simulink library "spsDiodeModel_R"  (R2023b)
settings: Solver=ode45  StartTime=0.0  StopTime=10.0  RelTol=1e-3
undefined symbols (not defined in the file): IC, Lon, Ron, Vf
settings Model: Creator=The MathWorks, Inc.  LastModifiedBy=rober
settings SolverCC: AlgebraicLoopSolver=TrustRegion
settings DataIOCC: LimitDataPoints=on  SaveFormat=Array  SignalLoggingSaveFormat=ModelDataLogs  ReturnWorkspaceOutputs=off
settings OptimizationCC: BlockReduction=off  BooleanDataType=off  ExpressionDepthLimit=2147483647  LifeSpan=inf
settings DebuggingCC: SaveWithParameterizedLinksMsg=none  UnderspecifiedInitializationDetection=Classic  MergeDetectMultiDrivingBlocksExec=none  SignalResolutionControl=TryResolveAllWithWarning  FcnCallInpInsideContextMsg=warning  UnconnectedInputMsg=warning  UnconnectedOutputMsg=warning  UnconnectedLineMsg=warning  StateNameClashWarn=warning  SFUnexpectedBacktrackingDiag=warning  SFNoUnconditionalDefaultTransitionDiag=warning  SFExecutionAtInitializationDiag=none  ArithmeticOperatorsInVariantConditions=warning
settings HardwareCC: ProdBitPerPointer=32  ProdBitPerSizeT=32  ProdBitPerPtrDiffT=32  ProdLargestAtomicFloat=None  ProdIntDivRoundTo=Undefined  ProdEndianess=Unspecified  ProdWordSize=32  ProdHWDeviceType=32-bit Generic  TargetUnknown=on
settings ModelReferenceCC: PropagateSignalLabelsOutOfModel=off
settings SFSimCC: SimUseLocalCustomCode=off  CustomCodeUndefinedFunction=UseInterfaceOnly
settings RTWCC: RTWUseLocalCustomCode=off
settings CodeAppCC: StateflowObjectComments=on
settings GRTTargetCC: TargetLangStandard=C89/C90 (ANSI)  CombineOutputUpdateFcns=off  GRTInterface=on
settings ConfigComp: CovMetricSettings=dw  CovSaveCumulativeToWorkspaceVar=on  CovSaveSingleToWorkspaceVar=on  CovExternalEMLEnable=off  CovSFcnEnable=off

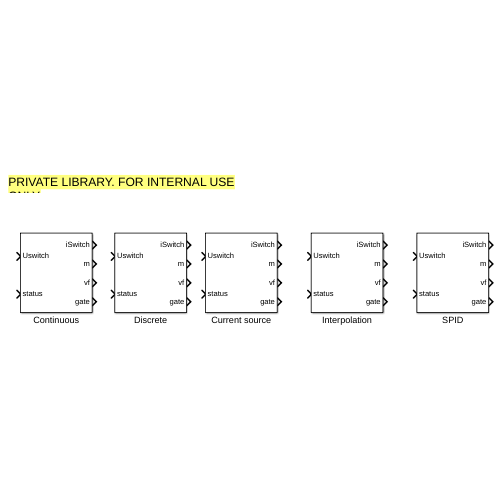
[thumbnail: Simulink's stored preview of the top-level diagram]
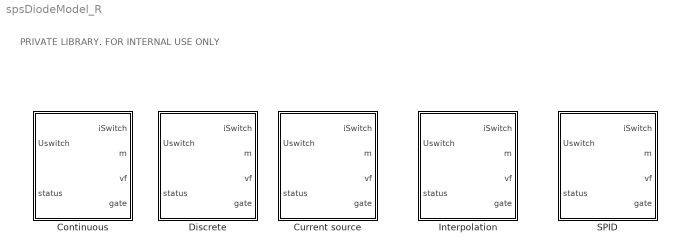
== system spsDiodeModel_R ==
  note: PRIVATE LIBRARY. FOR INTERNAL USE ONLY
  Continuous : Subsystem  mask(ContinuousModel){}
  Current source : Subsystem  mask(CurrentSourceDiode){}
  Discrete : Subsystem  mask(DiscreteModel){}
  Interpolation : Subsystem  mask(DiscreteModel){}
  SPID : Subsystem  mask(DiscreteModel){}

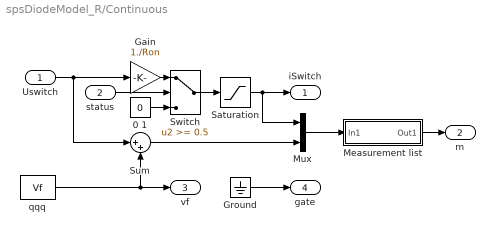
== system spsDiodeModel_R/Continuous ==
  Uswitch : Inport
  status : Inport  Port=2
  0 1 : Constant  Value=0
  Gain : Gain  Gain=1./Ron  SaturateOnIntegerOverflow=on  OutDataTypeStr=Inherit: Same as input  ParamDataTypeStr=Inherit: Same as input
  Ground : Ground
  Measurement list : Subsystem
  Mux : Mux  Inputs=2
  Saturation : Saturate  UpperLimit=inf  LowerLimit=0
  Sum : Sum  Inputs=|++  InputSameDT=on  SaturateOnIntegerOverflow=on  OutDataTypeStr=Inherit: Same as first input
  Switch : Switch  Threshold=0.5  SaturateOnIntegerOverflow=off
  qqq : Constant  Value=Vf
  iSwitch : Outport
  m : Outport  Port=2
  vf : Outport  Port=3
  gate : Outport  Port=4
  wires:
  Uswitch/1 -> Sum/1, Gain/1
  Gain/1 -> Switch/1
  0 1/1 -> Switch/3
  Switch/1 -> Saturation/1
  qqq/1 -> vf/1, Sum/2
  Saturation/1 -> Mux/1, iSwitch/1
  Sum/1 -> Mux/2
  Mux/1 -> Measurement list/1(In1)
  status/1 -> Switch/2
  Measurement list/1(Out1) -> m/1
  Ground/1 -> gate/1

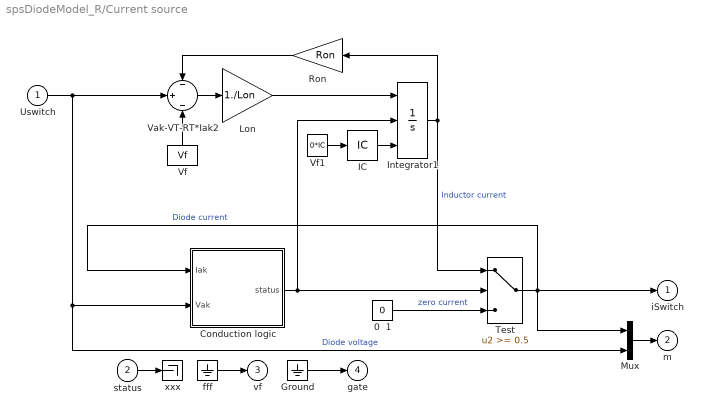
== system spsDiodeModel_R/Current source ==
  Uswitch : Inport
  status : Inport  Port=2
  0  1 : Constant  Value=0
  Conduction logic : Subsystem
  Ground : Ground
  IC : InitialCondition  Value=IC
  Integrator1 : Integrator  ExternalReset=rising  InitialConditionSource=external  LimitOutput=on  LowerSaturationLimit=0
  Lon : Gain  Gain=1./Lon  SaturateOnIntegerOverflow=on  OutDataTypeStr=Inherit: Same as input  ParamDataTypeStr=Inherit: Same as input
  Mux : Mux  Inputs=2
  Ron : Gain  Gain=Ron  SaturateOnIntegerOverflow=on  OutDataTypeStr=Inherit: Same as input  ParamDataTypeStr=Inherit: Same as input
  Test : Switch  Threshold=0.5  SaturateOnIntegerOverflow=off
  Vak-VT-RT*Iak2 : Sum  Inputs=-|+|-  InputSameDT=on  SaturateOnIntegerOverflow=on  OutDataTypeStr=Inherit: Same as first input
  Vf : Constant  Value=Vf
  Vf1 : Constant  Value=0*IC
  fff : Ground
  xxx : Terminator
  iSwitch : Outport  InitialOutput=0
  m : Outport  Port=2  InitialOutput=0
  vf : Outport  Port=3  InitialOutput=0
  gate : Outport  Port=4  InitialOutput=0
  wires:
  status/1 -> xxx/1
  fff/1 -> vf/1
  Test/1 -> Conduction logic/1(Iak), Mux/1, iSwitch/1  "Diode current"
  0  1/1 -> Test/3  "zero current"
  Vf1/1 -> IC/1
  Vf/1 -> Vak-VT-RT*Iak2/3
  Ron/1 -> Vak-VT-RT*Iak2/1
  Integrator1/1 -> Test/1, Ron/1  "Inductor current"
  Vak-VT-RT*Iak2/1 -> Lon/1
  Conduction logic/1(status) -> Test/2, Integrator1/2
  Lon/1 -> Integrator1/1
  IC/1 -> Integrator1/3
  Uswitch/1 -> Vak-VT-RT*Iak2/2, Conduction logic/2(Vak), Mux/2  "Diode voltage"
  Mux/1 -> m/1
  Ground/1 -> gate/1

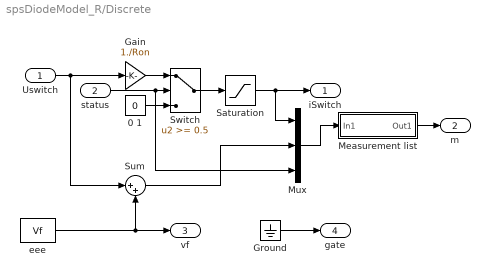
== system spsDiodeModel_R/Discrete ==
  Uswitch : Inport
  status : Inport  Port=2
  0 1 : Constant  Value=0
  Gain : Gain  Gain=1./Ron  SaturateOnIntegerOverflow=on  OutDataTypeStr=Inherit: Same as input  ParamDataTypeStr=Inherit: Same as input
  Ground : Ground
  Measurement list : Subsystem
  Mux : Mux  Inputs=3
  Saturation : Saturate  UpperLimit=inf  LowerLimit=0
  Sum : Sum  Inputs=|++  InputSameDT=on  SaturateOnIntegerOverflow=on  OutDataTypeStr=Inherit: Same as first input
  Switch : Switch  Threshold=0.5  SaturateOnIntegerOverflow=off
  eee : Constant  Value=Vf
  iSwitch : Outport
  m : Outport  Port=2
  vf : Outport  Port=3
  gate : Outport  Port=4
  wires:
  Measurement list/1(Out1) -> m/1
  status/1 -> Mux/3, Switch/2
  Mux/1 -> Measurement list/1(In1)
  Sum/1 -> Mux/2
  Saturation/1 -> iSwitch/1, Mux/1
  eee/1 -> vf/1, Sum/2
  Switch/1 -> Saturation/1
  0 1/1 -> Switch/3
  Gain/1 -> Switch/1
  Uswitch/1 -> Sum/1, Gain/1
  Ground/1 -> gate/1

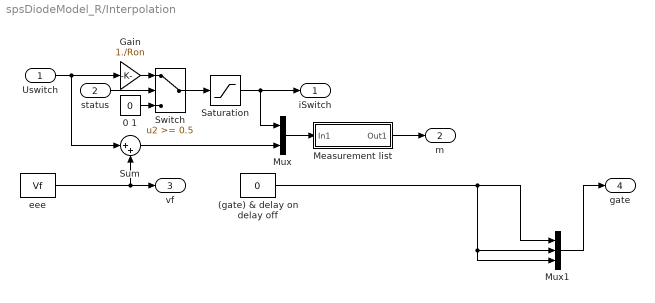
== system spsDiodeModel_R/Interpolation ==
  Uswitch : Inport
  status : Inport  Port=2
  (gate) & delay on delay off : Constant  Value=0
  0 1 : Constant  Value=0
  Gain : Gain  Gain=1./Ron  SaturateOnIntegerOverflow=on  OutDataTypeStr=Inherit: Same as input  ParamDataTypeStr=Inherit: Same as input
  Measurement list : Subsystem
  Mux : Mux  Inputs=2
  Mux1 : Mux  Inputs=3
  Saturation : Saturate  UpperLimit=inf  LowerLimit=0
  Sum : Sum  Inputs=|++  InputSameDT=on  SaturateOnIntegerOverflow=on  OutDataTypeStr=Inherit: Same as first input
  Switch : Switch  Threshold=0.5  SaturateOnIntegerOverflow=off
  eee : Constant  Value=Vf
  iSwitch : Outport
  m : Outport  Port=2
  vf : Outport  Port=3
  gate : Outport  Port=4
  wires:
  Uswitch/1 -> Sum/1, Gain/1
  Gain/1 -> Switch/1
  0 1/1 -> Switch/3
  Switch/1 -> Saturation/1
  eee/1 -> Sum/2, vf/1
  Saturation/1 -> Mux/1, iSwitch/1
  Sum/1 -> Mux/2
  Mux/1 -> Measurement list/1(In1)
  status/1 -> Switch/2
  Measurement list/1(Out1) -> m/1
  (gate) & delay on delay off/1 -> Mux1/3, Mux1/2, Mux1/1
  Mux1/1 -> gate/1

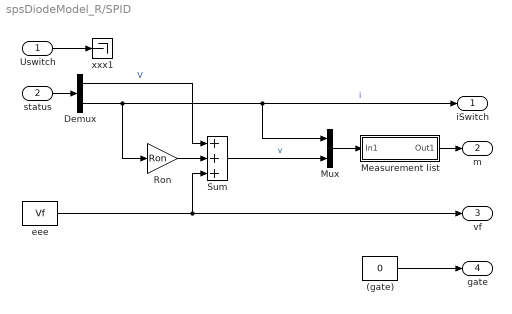
== system spsDiodeModel_R/SPID ==
  Uswitch : Inport
  status : Inport  Port=2
  (gate) : Constant  Value=0
  Demux : Demux  Outputs=2
  Measurement list : Subsystem
  Mux : Mux  Inputs=2
  Ron : Gain  Gain=Ron
  Sum : Sum  Inputs=+++  InputSameDT=on  SaturateOnIntegerOverflow=on  OutDataTypeStr=Inherit: Same as first input
  eee : Constant  Value=Vf
  xxx1 : Terminator
  iSwitch : Outport
  m : Outport  Port=2
  vf : Outport  Port=3
  gate : Outport  Port=4
  wires:
  (gate)/1 -> gate/1
  Measurement list/1(Out1) -> m/1
  Mux/1 -> Measurement list/1(In1)
  eee/1 -> vf/1, Sum/3
  status/1 -> Demux/1
  Demux/1 -> Sum/1  "V"
  Demux/2 -> iSwitch/1, Mux/1, Ron/1  "i"
  Sum/1 -> Mux/2  "v"
  Ron/1 -> Sum/2
  Uswitch/1 -> xxx1/1

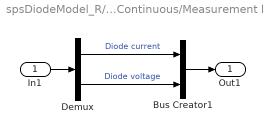
== system spsDiodeModel_R/Continuous/Measurement list ==
  In1 : Inport
  Bus Creator1 : BusCreator  Inputs=2
  Demux : Demux  Outputs=[1,1]
  Out1 : Outport
  wires:
  In1/1 -> Demux/1
  Bus Creator1/1 -> Out1/1
  Demux/1 -> Bus Creator1/1  "Diode current"
  Demux/2 -> Bus Creator1/2  "Diode voltage"

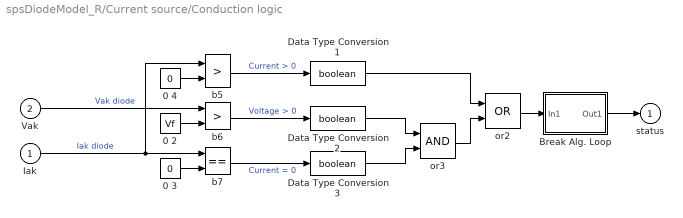
== system spsDiodeModel_R/Current source/Conduction logic ==
  Iak : Inport
  Vak : Inport  Port=2
  0 2 : Constant  Value=Vf
  0 3 : Constant  Value=0
  0 4 : Constant  Value=0
  Break Alg. Loop : Subsystem  mask{Nsw=length(Lon), IC=IC}
      mask prompts: Nsw "number of switches"; IC "Initial condition"
  Data Type Conversion1 : DataTypeConversion  OutDataTypeStr=boolean
  Data Type Conversion2 : DataTypeConversion  OutDataTypeStr=boolean
  Data Type Conversion3 : DataTypeConversion  OutDataTypeStr=boolean
  b5 : RelationalOperator  Operator=>
  b6 : RelationalOperator  Operator=>
  b7 : RelationalOperator  Operator===
  or2 : Logic  Operator=OR
  or3 : Logic
  status : Outport  InitialOutput=0
  wires:
  Data Type Conversion3/1 -> or3/2
  Data Type Conversion2/1 -> or3/1
  Data Type Conversion1/1 -> or2/1
  Break Alg. Loop/1(Out1) -> status/1
  Iak/1 -> b7/1, b5/1  "Iak diode"
  b7/1 -> Data Type Conversion3/1  "Current = 0"
  b5/1 -> Data Type Conversion1/1  "Current > 0"
  0 4/1 -> b5/2
  or2/1 -> Break Alg. Loop/1(In1)
  or3/1 -> or2/2
  b6/1 -> Data Type Conversion2/1  "Voltage > 0"
  0 2/1 -> b6/2
  0 3/1 -> b7/2
  Vak/1 -> b6/1  "Vak diode"

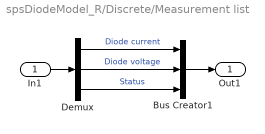
== system spsDiodeModel_R/Discrete/Measurement list ==
  In1 : Inport
  Bus Creator1 : BusCreator  Inputs=3
  Demux : Demux  Outputs=[1,1,1]
  Out1 : Outport
  wires:
  Demux/2 -> Bus Creator1/2  "Diode voltage"
  Demux/1 -> Bus Creator1/1  "Diode current"
  Bus Creator1/1 -> Out1/1
  In1/1 -> Demux/1
  Demux/3 -> Bus Creator1/3  "Status"

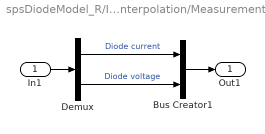
== system spsDiodeModel_R/Interpolation/Measurement list ==
  In1 : Inport
  Bus Creator1 : BusCreator  Inputs=2
  Demux : Demux  Outputs=[1,1]
  Out1 : Outport
  wires:
  In1/1 -> Demux/1
  Bus Creator1/1 -> Out1/1
  Demux/1 -> Bus Creator1/1  "Diode current"
  Demux/2 -> Bus Creator1/2  "Diode voltage"

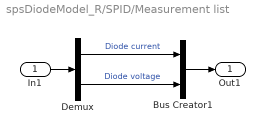
== system spsDiodeModel_R/SPID/Measurement list ==
  In1 : Inport
  Bus Creator1 : BusCreator  Inputs=2
  Demux : Demux  Outputs=[1,1]
  Out1 : Outport
  wires:
  Demux/2 -> Bus Creator1/2  "Diode voltage"
  Demux/1 -> Bus Creator1/1  "Diode current"
  Bus Creator1/1 -> Out1/1
  In1/1 -> Demux/1

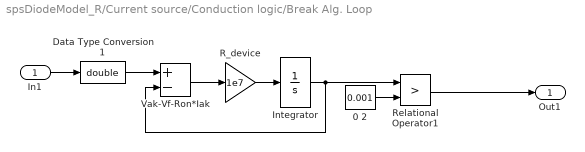
== system spsDiodeModel_R/Current source/Conduction logic/Break Alg. Loop ==
  In1 : Inport
  0 2 : Constant  Value=0.001
  Data Type Conversion1 : DataTypeConversion  OutDataTypeStr=double
  Integrator : Integrator  InitialCondition=0.00101*(IC&1)  LimitOutput=on  UpperSaturationLimit=0.00101
  R_device : Gain  Gain=1e7  SaturateOnIntegerOverflow=on  OutDataTypeStr=Inherit: Same as input  ParamDataTypeStr=Inherit: Same as input
  Relational Operator1 : RelationalOperator  Operator=>
  Vak-Vf-Ron*Iak : Sum  Inputs=+-  InputSameDT=on  SaturateOnIntegerOverflow=on  OutDataTypeStr=Inherit: Same as first input
  Out1 : Outport
  wires:
  Relational Operator1/1 -> Out1/1
  0 2/1 -> Relational Operator1/2
  Integrator/1 -> Relational Operator1/1, Vak-Vf-Ron*Iak/2
  Vak-Vf-Ron*Iak/1 -> R_device/1
  R_device/1 -> Integrator/1
  Data Type Conversion1/1 -> Vak-Vf-Ron*Iak/1
  In1/1 -> Data Type Conversion1/1
